simulink model "StaticCalc_TestBed"  (R2015a)
settings: Solver=FixedStepDiscrete  StartTime=0.0  StopTime=1  FixedStep=1  RelTol=1e-3
undefined symbols (not defined in the file): MWS
libraries: Lib_Turbo_StaticCalc_TMATS x1
settings Model: Creator=jwchapm2  LastModifiedBy=jwchapm2
settings OptimizationCC: ExpressionDepthLimit=2147483647
settings DebuggingCC: UnderspecifiedInitializationDetection=Classic  MergeDetectMultiDrivingBlocksExec=none  SolverPrmCheckMsg=warning  StateNameClashWarn=warning

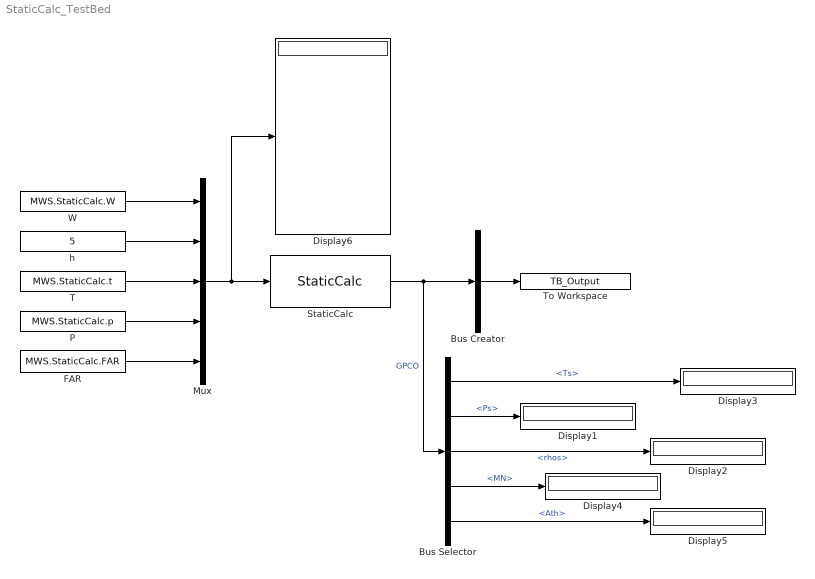
== system StaticCalc_TestBed ==
  Bus Selector : BusSelector  OutputSignals=Ts,Ps,rhos,MN,Ath
  Bus Creator : BusCreator  Inputs=1
  Display{1..6} (6 alike) : Display
  FAR : Constant  Value=MWS.StaticCalc.FAR
  Mux : Mux  Inputs=5
  P : Constant  Value=MWS.StaticCalc.p
  StaticCalc : Lib_Turbo_StaticCalc_TMATS/StaticCalc  ST_M=off  Ath_M=MWS.StaticCalc.Ath  MN_M=MWS.StaticCalc.MN  X_FARVec_M=[0; 0.0050; 0.0100; 0.0150; 0.0200; 0.0250; 0.0300]  Y_TtVec_M=[300 10000]  T_RtArray_M="[0.0686;    0.0686;    0.0686;    0.0686;    0.0686;    0.0686;    0.0686]"  T_gammaArray_M=[ 1.4 1.4 1.4 1.4 1.4 1.4 1.4; 1.4 1.4 1.4 1.4 1.4 1.4 1.4]
  T : Constant  Value=MWS.StaticCalc.t
  To Workspace : ToWorkspace  VariableName=TB_Output  SampleTime=-1
  W : Constant  Value=MWS.StaticCalc.W
  h : Constant  Value=5
  wires:
  FAR/1 -> Mux/5
  StaticCalc/1 -> Bus Selector/1, Bus Creator/1  "GPCO"
  Bus Creator/1 -> To Workspace/1
  P/1 -> Mux/4
  T/1 -> Mux/3
  W/1 -> Mux/1
  h/1 -> Mux/2
  Mux/1 -> Display6/1, StaticCalc/1
  Bus Selector/1 -> Display3/1  "<Ts>"
  Bus Selector/2 -> Display1/1  "<Ps>"
  Bus Selector/3 -> Display2/1  "<rhos>"
  Bus Selector/4 -> Display4/1  "<MN>"
  Bus Selector/5 -> Display5/1  "<Ath>"
